simulink model "openloop_simulink"  (R2020b)
settings: Solver=VariableStepAuto  StartTime=0.0  StopTime=1  RelTol=1e-3
values from neighbouring files (symbols this model uses):
  b = Trated / (Wrated * 2*pi / 60)    (= 0.0130454871387)    [closedloop_mat.m]    (also in openloop_mat.m)
  J = 0.0000071    (= 7.1e-06)    [closedloop_mat.m]    (also in openloop_mat.m)
  km = 0.0458    [closedloop_mat.m]    (also in openloop_mat.m)
  Lf = 2.63E-3    (= 0.00263)    [closedloop_mat.m]    (also in openloop_mat.m)
  n = 11.5    [closedloop_mat.m]    (also in openloop_mat.m)
  Rf = 2.49    [closedloop_mat.m]    (also in openloop_mat.m)
settings Model: Creator=Kevin Rim  LastModifiedBy=Kevin Rim

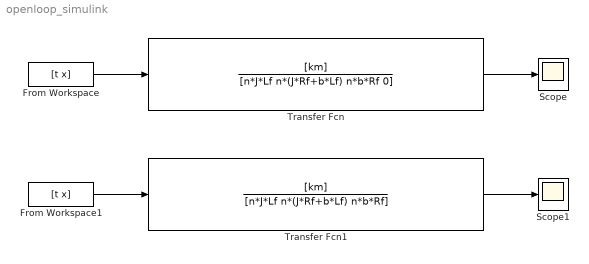
== system openloop_simulink ==
  From Workspace : FromWorkspace  VariableName=[t x]  SampleTime=-1
  From Workspace1 : FromWorkspace  VariableName=[t x]  SampleTime=-1
  Scope : Scope
  Scope1 : Scope
  Transfer Fcn : TransferFcn  Numerator=[km]  Denominator=[n*J*Lf n*(J*Rf+b*Lf) n*b*Rf 0]
  Transfer Fcn1 : TransferFcn  Numerator=[km]  Denominator=[n*J*Lf n*(J*Rf+b*Lf) n*b*Rf]
  wires:
  From Workspace/1 -> Transfer Fcn/1
  Transfer Fcn/1 -> Scope/1
  From Workspace1/1 -> Transfer Fcn1/1
  Transfer Fcn1/1 -> Scope1/1
